simulink subsystem "Day4_5_Scenario_1"  (R2024a)
settings: Solver=VariableStepAuto  StartTime=0.0  StopTime=10.0  RelTol=1e-3
libraries: CarMaker4SL x29, robotalgslib x1, matrix_library x1, slpidlib x1
(part 2 of 2)

== matlab function Day4_5_Scenario_1/Function-Call Subsystem1/MATLAB Function ==
  data: currPoseRear input; v input; waypoints input; delta output
function delta = lateral_spp_controller(currPoseRear, v, waypoints)
%▴ Hybrid Stanley & Pure Pursuit + Monotonic Index Enforcement
% Inputs:
%   currPoseRear : [x_rear; y_rear; psi] (후륜축 기준 위치 및 자세)
%   v            : 현재 속도 (m/s)
%   waypoints    : N×3 [x_i, y_i, psi_i] (경로 웨이포인트)
% Output:
%   delta        : 전륜 조향각 (rad)

    %#codegen
    %% persistent 변수 초기화
    persistent idx_last delta_prev
    if isempty(idx_last)
        idx_last   = 1;    % 마지막 타겟 인덱스 (초기값)
    end
    if isempty(delta_prev)
        delta_prev = 0;    % 이전 조향각 (로우패스 필터용)
    end

    %% 파라미터
    L        = 2.9;                             % 휠베이스 [m]
    k_st     = 1.0;                             % Stanley 이득
    eps_v    = 0.1;                             % 속도 안정화 상수
    deltaMax = deg2rad(40);                     % 최대 조향각 제한 ±40°
    e_thresh = 0.5;                             % SPP 전환 임계값 [m]
    k_pp     = 0.3;                             % 룩어헤드 속도 이득
    Ld_min   = 2.0;                             % 룩어헤드 최솟값 [m]
    Ld_max   = 4.0;                             % 룩어헤드 최댓값 [m]
    alpha_f  = 0.35;                            % 로우패스 필터 상수

    %% 전륜축 위치 계산 (후륜축 기준 → 전륜축 좌표 변환)
    x_f = currPoseRear(1) + L*cos(currPoseRear(3));
    y_f = currPoseRear(2) + L*sin(currPoseRear(3));

    %% 전방 웨이포인트만 선별 (로컬 좌표계)
    psi_wrapped = wrapToPi(currPoseRear(3));    % yaw를 –π~π로 유지
    heading_vec = [cos(psi_wrapped), sin(psi_wrapped)];
    diffs       = waypoints(:,1:2) - currPoseRear(1:2)';
    forward_idx = find(diffs * heading_vec' > 0);  % 전방 idx
    if isempty(forward_idx)
        forward_idx = (1:size(waypoints,1))';       % 전방이 없으면 전체 사용
    end

    %% 룩어헤드 거리 계산
    Ld_raw = k_pp * v + eps_v;
    Ld     = min(max(Ld_raw, Ld_min), Ld_max);

    %% 후보 인덱스 범위 설정 (룩어헤드 윈도우)
    N = size(waypoints,1);
    extra     = round(0.2 * Ld);                  % 윈도우 여분
    start_idx = max(idx_last - extra, 1);
    end_idx   = min(idx_last + round(Ld) + extra, N);
    cand_idx  = intersect(forward_idx, (start_idx:end_idx)');

    if isempty(cand_idx)
        cand_idx = forward_idx;  % 후보 없으면 전방 전체 사용
    end

    %% 최단거리 웨이포인트 선택
    dists = hypot(waypoints(cand_idx,1)-x_f, waypoints(cand_idx,2)-y_f);
    [~, rel] = min(dists);
    idx_new  = cand_idx(rel);  % 새로 계산된 인덱스

    %% 1) Monotonic Index Enforcement 적용
    % 새 인덱스(idx_new)가 이전 idx_last보다 작으면 무시
    if idx_new < idx_last
        idx_last = idx_last;    % 변경 없이 유지
    else
        idx_last = idx_new;     % 증가 시에만 갱신
    end

    %% 참조점 정보 추출
    x_ref   = waypoints(idx_last,1);
    y_ref   = waypoints(idx_last,2);
    psi_ref = waypoints(idx_last,3);

    %% Heading error 및 Cross-Track error 계산
    theta_e = wrapToPi(psi_ref - currPoseRear(3));  
    e_cte   = -(x_f - x_ref)*sin(psi_ref) + (y_f - y_ref)*cos(psi_ref);

    %% 제어 분기: Pure Pursuit vs Stanley
    if abs(e_cte) > e_thresh
        % Pure Pursuit
        alpha     = wrapToPi(atan2(y_ref-currPoseRear(2), x_ref-currPoseRear(1)) ...
                     - currPoseRear(3));
        delta_cmd = atan2(2 * L * sin(alpha), Ld);
    else
        % Stanley
        delta_cmd = theta_e + atan((k_st * e_cte) / (v + eps_v));
    end

    %% 로우패스 필터 적용 및 조향각 포화
    delta       = alpha_f * delta_cmd + (1 - alpha_f) * delta_prev;
    delta_prev  = delta;  
    delta       = max(min(delta, deltaMax), -deltaMax);

end

== matlab function Day4_5_Scenario_1/MATLAB Function4  ==
  settings: updateMethod=DISCRETE  sampleTime=0.05
  data: path input; local_waypoints_ output; vehicle_position input; head input
function local_waypoints_ = global_to_local_waypoints(path, vehicle_position, head)
    %#codegen
    % 글로벌 경로를 로컬 경로로 변환해주는 함수
    % path : [x, y, yaw] (경로 점들)
    % vehicle_position : [Ego_Global_X, Ego_Global_Y]
    % head : Ego_Yaw (rad)
    % 출력: 로컬 좌표 (x_local, y_local, yaw_local)

    % 최대 경로 점 개수 설정
    max_points = 100;

    % 초기화
    local_waypoints_ = NaN(max_points, 3);  % 고정 크기 배열

    % 차량 위치 및 헤딩 추출
    ego_x = vehicle_position(1);
    ego_y = vehicle_position(2);
    ego_yaw = head;

    % 회전 행렬 생성 (글로벌→로컬 변환)
    R = [cos(-ego_yaw) -sin(-ego_yaw); 
         sin(-ego_yaw)  cos(-ego_yaw)];

    count = int32(0);  % 경로 점 개수

    % 각 경로 포인트에 대해 변환 수행
    for i = 1:min(size(path, 1), max_points)
        % 글로벌 좌표에서 차량까지의 상대 위치
        dx = path(i, 1) - ego_x;  % X 좌표 차이
        dy = path(i, 2) - ego_y;  % Y 좌표 차이

        % 회전 변환 적용
        local_pos = R * [dx; dy];
        
        % Yaw 변환: 로컬 좌표계에서의 Yaw
        global_yaw = path(i, 3);
        local_yaw = wrapToPi(global_yaw - ego_yaw);  % 로컬 yaw 변환

        % 차량으로부터 waypoint까지의 거리
        distance = sqrt(local_pos(1)^2 + local_pos(2)^2);

        % 첫 번째 유효 경로 점 저장 (x > 0인 첫 포인트)
        if count == 0 && local_pos(1) > 0
            count = count + 1;
            local_waypoints_(count, :) = [local_pos(1), local_pos(2), local_yaw];
        end

        % 유효 조건 만족 시 좌표 저장
        % 1. x 좌표가 0보다 큰 경우
        % 2. 이전 x 좌표보다 큰 경우
        % 3. 차량으로부터 30m 이내인 경우
        % 4. 로컬 x값이 증가하는 방향인 경우
        if count ~= 0 && local_pos(1) > 0 && local_pos(1) > local_waypoints_(count, 1) && distance < 30
            % 고정 크기 초과 방지
            if count < max_points
                count = count + 1;
                local_waypoints_(count, :) = [local_pos(1), local_pos(2), local_yaw];
            else
                warning('Maximum number of waypoints reached.');
                break;
            end
        end
    end

    % 남은 부분을 NaN으로 채움
    if count < max_points
        local_waypoints_((count+1):max_points, :) = NaN;
    end
end

== matlab function Day4_5_Scenario_1/Function-Call Subsystem/MATLAB Function1 ==
  settings: sampleTime=0.05
  data: map_boundary input; mapMatrix output size=[1000, 1000]; traffic_info input; traffic_size input
% map_boundary = [0, 0, 100, 0, 100, -100, 0, -100];  % 시계방향 사각형
% traffic_info = [
%     40   -12   pi/2;
%     40   -24   pi/2;
%     40   -36   pi/2;
%     40   -48   pi/2;
%     39   -50   0;
%     51   -50   0;
%     63   -50   0];  % [x_head, y_head, yaw]
% traffic_size = [2.48, 11.5];    % [width, length] (m)
% start_point  = [0, -20];
% finish_point = [80, -3];
% 
% a = generate_map_(map_boundary, traffic_info, traffic_size);

function mapMatrix = generate_map_(map_boundary, traffic_info, traffic_size)
%#codegen
% 맵 바운더리 + 장애물 테두리를 마스킹하는 함수
% Y축 반전 처리만 적용 (Y는 -100~0 → mapMatrix는 1~100)

    % === 초기화 ===
    mapMatrix = zeros(100, 100);

    % === reshape 및 파라미터 ===
    traffic_info = reshape(traffic_info, [], 3);  % [N x 3]
    num_traffic = size(traffic_info, 1);
    width  = traffic_size(1);
    length = traffic_size(2);

    % === 장애물 테두리 처리 ===
    for i = 1:num_traffic
        x_head = traffic_info(i,1);
        y_head = traffic_info(i,2);
        yaw    = traffic_info(i,3);
       
        % 머리 좌표를 중심 기준으로 사용
        xc = x_head;
        yc = y_head;

        dx = width / 2;
        dy = length;
        local = [
            0, -dx;
            0,  dx;
            dy, dx;
            dy, -dx
        ];

        R = [cos(yaw), -sin(yaw); sin(yaw), cos(yaw)];
        global_pts = zeros(5, 2);  % 4개 꼭짓점 + 첫 점
        
        global_pts(1:4, :) = (R * local')' + [xc, yc];
        global_pts(5, :)   = global_pts(1, :);  % 꼭짓점 닫기

        for k = 1:4
            x1 = global_pts(k,1);   y1 = global_pts(k,2);
            x2 = global_pts(k+1,1); y2 = global_pts(k+1,2);
            N = 100;
            xs = linspace(x1, x2, N);
            ys = linspace(y1, y2, N);
            for j = 1:N
                x_idx = round(xs(j));
                y_idx = round(-ys(j));  % ✅ Y 좌표 반전

                % 인덱스 클리핑
                x_idx = min(max(x_idx, 1), 100);
                y_idx = min(max(y_idx, 1), 100);

                mapMatrix(y_idx, x_idx) = 1;
            end
        end
    end

    % === 바운더리 테두리 처리 ===
    xb = map_boundary(1:2:end);
    yb = map_boundary(2:2:end);
    xb(end+1) = xb(1);
    yb(end+1) = yb(1);
    for k = 1:4
        x1 = xb(k);   y1 = yb(k);
        x2 = xb(k+1); y2 = yb(k+1);
        N = 100;
        xs = linspace(x1, x2, N);
        ys = linspace(y1, y2, N);
        for j = 1:N
            x_idx = round(xs(j));
            y_idx = round(-ys(j));  % ✅ Y 좌표 반전

            % 인덱스 클리핑
            x_idx = min(max(x_idx, 1), 100);
            y_idx = min(max(y_idx, 1), 100);

            mapMatrix(y_idx, x_idx) = 1;
        end
    end
end

== stateflow chart Day4_5_Scenario_1/Chart1 ==
  settings: updateMethod=DISCRETE  sampleTime=0.05
  state drawMap
    entry:
    draw_Map();
  state goParking
    during:
    go_Parking();
  (default) -> drawMap
  drawMap -> goParking : after(10,tick)
  events: go_Parking output FUNCTION_CALL_EVENT; draw_Map output FUNCTION_CALL_EVENT

== matlab function Day4_5_Scenario_1/Function-Call Subsystem/MATLAB Function4 ==
  data: start input; goal input; obstacle_list input; path output
function path = hybrid_astar_(start, goal, obstacle_list)
%#codegen
disp('start hybrid a*');
% 기본 파라미터 설정
R = 4;
Vx = 3;
delta_time_step = 1;
weight = 1.3;
space = [0, 100, -100, 0];
res_dijkstra = 1;

% 경로 배열 초기화 (고정 크기)
path = NaN(100, 3);  % 고정 크기 배열
path_count = int32(0);

% 구조체 초기화 함수
default_node = struct('position', zeros(1,3), 'heading', 0.0, 'g', 0.0, 'h', 0.0, 'f', 0.0, 'parent', int32(0));
open_list = repmat(default_node, 1, 100);
closed_list = repmat(default_node, 1, 10000);

% Dijkstra를 이용한 비용 맵 생성
cost_map = run_dijkstra(goal, obstacle_list, space, res_dijkstra);
start_node = create_node(int32(0), start);
goal_node = create_node(int32(0), goal);

% 초기화
open_list(1) = start_node;
open_count = int32(1);
closed_count = int32(0);

% Hybrid A* 알고리즘
while open_count > 0
    % 최저 비용 노드 선택
    f_values = arrayfun(@(n) n.f, open_list(1:open_count));
    [~, idx] = min(f_values);
    temp_node = open_list(idx);
    open_list(idx) = open_list(open_count);
    open_count = open_count - 1;
    closed_count = closed_count + 1;
    closed_list(closed_count) = temp_node;

    % 목표 도달 확인
    if isSamePosition(temp_node, goal_node, 5)
         % — 첫 번째 행에 정확한 목표 지점(Finish_Point) 저장 —
        path_count = int32(1);               % 인덱스 1로 초기화
        path(path_count, :) = goal;         % goal [x, y, yaw] 저장

        % — Finish_Point 이후로 역추적된 노드들 저장 —
        while temp_node.parent > 0 && path_count < 100
            path_count = path_count + 1;    % 다음 인덱스
            path(path_count, :) = temp_node.position;  % 노드 위치 저장
            parent_idx     = temp_node.parent;         % 부모 인덱스
            temp_node      = closed_list(parent_idx);  % 부모 노드로 이동
        end

        % — 나머지 행은 NaN으로 채워서 크기 고정 유지 —
        if path_count < 100
            path((path_count+1):100, :) = NaN;
        end
        return;  % 완성된 path 반환
    end

    % 가능한 액션 생성 및 탐색
    actions = get_action(R, Vx, delta_time_step);
    for i = 1:size(actions, 1)
        yaw_rate = actions(i, 1);
        dt = actions(i, 2);
        new_pos = vehicle_move(temp_node.position, yaw_rate, dt, Vx);
        
        % 탐색 공간 확인 및 충돌 검사
        if isNotInSearchingSpace(new_pos, space), continue; end
        if collision_check(temp_node.position, yaw_rate, dt, obstacle_list, Vx, space), continue; end
        
        % 자식 노드 생성
        child_node = create_node(closed_count, new_pos);
        if any(arrayfun(@(n) isSamePosition(n, child_node, 5) && isSameYaw(n, child_node, 0.3), closed_list(1:closed_count))), continue; end
        
        % 비용 계산
        yaw_diff = abs(angdiff(temp_node.heading, child_node.heading));
        turn_penalty = 2 * yaw_diff;
        child_node.g = temp_node.g + Vx * dt + turn_penalty;
        child_node.h = heuristic(child_node, goal_node, cost_map, space, res_dijkstra);
        child_node.f = child_node.g + weight * child_node.h;

        % 중복 노드 체크
        skip = false;
        for j = 1:open_count
            temp_open = open_list(j);
            if isSamePosition(temp_open, child_node, 5) && child_node.f >= temp_open.f
                skip = true; break;
            end
        end
        if skip, continue; end

        % 오픈 리스트에 추가
        open_count = open_count + 1;
        open_list(open_count) = child_node;
    end
end
% 경로 크기 고정으로 반환
path = path(1:100, :);
disp('return Path in hybrid a*');
end

% 노드 생성 함수
function node = create_node(parent, position)
    % 구조체 필드 초기화 고정
    node = struct('position', zeros(1,3), 'heading', 0.0, 'g', 0.0, 'h', 0.0, 'f', 0.0, 'parent', int32(parent));
    node.position = reshape(position, [1,3]);  % 강제로 크기 고정
    node.heading = position(3);
end

function h = heuristic(cur_node, goal_node, cost_map, space, res)
    gx = round((cur_node.position(1) - space(1)) / res) + 1;
    gy = round((cur_node.position(2) - space(3)) / res) + 1;
    [ny, nx] = size(cost_map);
    if gx < 1 || gx > nx || gy < 1 || gy > ny, h = 1e6; return; end
    cost_dijkstra = cost_map(gy, gx);
    dyaw = abs(angdiff(cur_node.heading, goal_node.heading));
    h = cost_dijkstra + 3 * dyaw;
end

function cost_map = run_dijkstra(goal, obstacle_list, space, res)
x_range = space(1):res:space(2);
y_range = space(3):res:space(4);
nx = length(x_range); ny = length(y_range);
cost_map = inf(ny, nx); visited = false(ny, nx);
gx = round((goal(1) - space(1)) / res) + 1;
gy = round((goal(2) - space(3)) / res) + 1;
cost_map(gy, gx) = 0;

% Preallocate the queue with a fixed size
q = zeros(10000, 2);
q_count = 1;
q(1, :) = [gx, gy];

while q_count > 0
    [~, idx] = min(cost_map(sub2ind(size(cost_map), q(1:q_count,2), q(1:q_count,1))));
    current = q(idx, :);
    q(idx, :) = q(q_count, :);
    q_count = q_count - 1;
    x = current(1); y = current(2);
    if visited(y, x), continue; end
    visited(y, x) = true;
    for dx = -1:1
        for dy = -1:1
            if dx == 0 && dy == 0, continue; end
            nx_ = x + dx; ny_ = y + dy;
            if nx_ < 1 || ny_ < 1 || nx_ > nx || ny_ > ny, continue; end
            px = space(1) + (nx_-1) * res;
            py = space(3) + (ny_-1) * res;
            in_collision = false;
            for k = 1:size(obstacle_list,1)
                if hypot(px - obstacle_list(k,1), py - obstacle_list(k,2)) < obstacle_list(k,3)
                    in_collision = true; break;
                end
            end
            if in_collision, continue; end
            cost = cost_map(y,x) + res * hypot(dx, dy);
            if cost < cost_map(ny_, nx_)
                cost_map(ny_, nx_) = cost;
                q_count = q_count + 1;
                q(q_count, :) = [nx_, ny_];
            end
        end
    end
end
end

function actions = get_action(R, Vx, delta_time_step)
    yaw_rate = Vx / R;
    distance_travel = Vx * delta_time_step;
    actions = [
        yaw_rate, delta_time_step, distance_travel;
       -yaw_rate, delta_time_step, distance_travel;
        yaw_rate/2, delta_time_step, distance_travel;
       -yaw_rate/2, delta_time_step, distance_travel;
        0.0, delta_time_step, distance_travel
    ];
end

function new_pos = vehicle_move(pos, yaw_rate, delta_time, Vx)
    x = pos(1); y = pos(2); yaw = pos(3);
    if abs(yaw_rate) > 1e-3
        R = Vx / yaw_rate;
        cx = x - R * sin(yaw);
        cy = y + R * cos(yaw);
        dtheta = yaw_rate * delta_time;
        x_new = cx + R * sin(yaw + dtheta);
        y_new = cy - R * cos(yaw + dtheta);
        yaw_new = yaw + dtheta;
    else
        x_new = x + Vx * delta_time * cos(yaw);
        y_new = y + Vx * delta_time * sin(yaw);
        yaw_new = yaw;
    end
    yaw_new = mod(yaw_new, 2*pi);
    new_pos = [x_new, y_new, yaw_new];
end

function is_collision = collision_check(pos, yaw_rate, dt, obs_list, Vx, space)
    new_pos = vehicle_move(pos, yaw_rate, dt, Vx);
    x = new_pos(1); y = new_pos(2);
    if x < space(1) || x > space(2) || y < space(3) || y > space(4)
        is_collision = true; disp('Out of boundary'); return;
    end
    is_collision = false;
    for i = 1:size(obs_list,1)
        dx = x - obs_list(i,1); dy = y - obs_list(i,2);
        if hypot(dx, dy) < obs_list(i,3)
            is_collision = true; 
            %disp('collision');
            return;
        end
    end
end

function same = isSamePosition(node1, node2, epsilon)
    dx = node1.position(1) - node2.position(1);
    dy = node1.position(2) - node2.position(2);
    same = hypot(dx, dy) < epsilon;
end

function same = isSameYaw(node1, node2, epsilon)
    dyaw = abs(wrapToPi(node1.heading - node2.heading));
    same = dyaw < epsilon;
end

function out = isNotInSearchingSpace(pos, space)
    x = pos(1); y = pos(2);
    out = ~(space(1) <= x && x <= space(2) && space(3) <= y && y <= space(4));
end

== matlab function Day4_5_Scenario_1/MATLAB Function5 ==
  settings: updateMethod=DISCRETE  sampleTime=0.05
  data: local_waypoints input; poly_coeff output
function poly_coeff = fit_polynomial_to_waypoints(local_waypoints)
    % waypoint를 curve fitting 한 다항식 계수 반환
    % input: 로컬 좌표 웨이포인트
    % output: 다항식 계수 (3차)

    % 웨이포인트 추출
    x_points = local_waypoints(:, 1);  % 로컬 x 좌표
    y_points = local_waypoints(:, 2);  % 로컬 y 좌표

    % 유효한 웨이포인트만 사용 (x 좌표가 양수인 것만)
    valid_indices = x_points > 0;
    x_valid = x_points(valid_indices);
    y_valid = y_points(valid_indices);

    % 웨이포인트가 충분한지 확인
    if length(x_valid) < 4
        % 웨이포인트가 부족하면 직선 경로 반환
        poly_coeff = [0, 0, 0, 0];  % y = 0 (직선)
    else
        % 3차 다항식 피팅 (y = ax^3 + bx^2 + cx + d)
        poly_coeff = polyfit(x_valid, y_valid, 3);
    end
end
